simulink model "ACAC2024A"  (R2023b)
settings: Solver=ode23tb  StartTime=0.0  StopTime=0.3  FixedStep=1e-6  RelTol=1e-2
libraries: spsIGBTDiodeLib x8, spsSeriesRLCBranchLib x5, spsCurrentMeasurementLib x4, spsVoltageMeasurementLib x4, spsGroundLib x2, slpidlib x2, spsTriangleGeneratorLib x2, spsACVoltageSourceLib x1, sps_lib x1
settings Model: Creator=yaoya  LastModifiedBy=yaoya

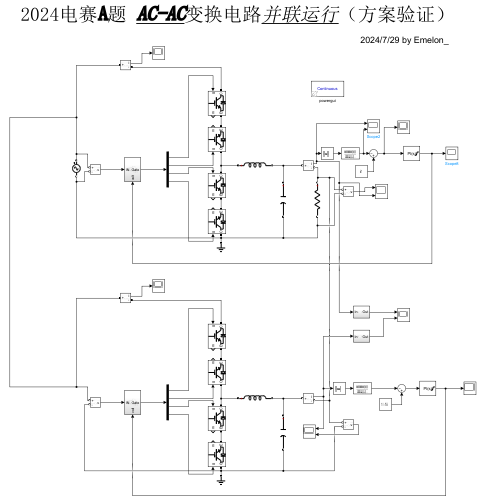
[thumbnail: Simulink's stored preview of the top-level diagram]
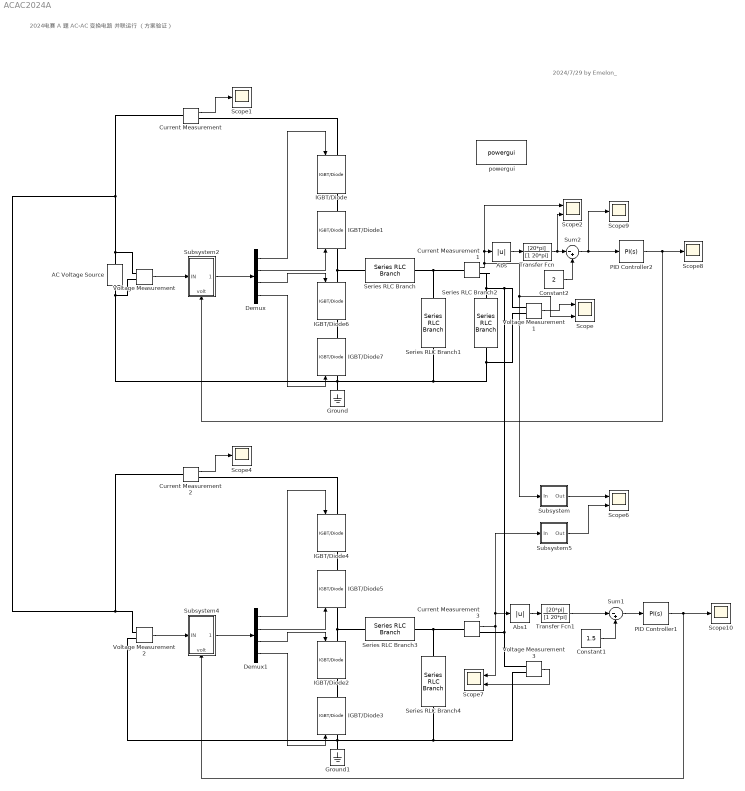
== system ACAC2024A ==
  note: 2024电赛 A 题 AC-AC 变换电路 并联运行 （方案验证）
  note: 2024/7/29 by Emelon_
  AC Voltage Source : spsACVoltageSourceLib/AC Voltage Source  Amplitude=100  Phase=0  Frequency=50  SampleTime=0  Measurements=None  BusType=swing  Pref=10e3  Qref=0  Qmin=-inf  Qmax=+inf
  Abs : Abs  SaturateOnIntegerOverflow=off
  Abs1 : Abs  SaturateOnIntegerOverflow=off
  Constant1 : Constant  Value=1.5
  Constant2 : Constant  Value=2
  Current Measurement{,1..3} (4 alike) : spsCurrentMeasurementLib/Current Measurement  PhasorSimulation=off  OutputType=Complex  PSBequivalent=0
  Demux : Demux
  Demux1 : Demux
  Ground : spsGroundLib/Ground  LConnTagsString=a
  Ground1 : spsGroundLib/Ground  LConnTagsString=a
  IGBT/Diode{,1..7} (8 alike) : spsIGBTDiodeLib/IGBT//Diode  Ron=1e-3  Rs=1e5  Cs=inf  Measurements=on
  PID Controller1 : slpidlib/PID Controller  Controller=PI  Form=Parallel  TimeDomain=Continuous-time  UseExternalTs=off  SampleTime=-1  IntegratorMethod=Forward Euler  FilterMethod=Forward Euler  ControllerParametersSource=internal  P=0.1  I=400  UseKiTs=off  D=10  N=100  UseFilter=on  TunerSelectOption=Transfer Function Based (PID Tuner App)  InitialConditionSource=internal  InitialConditionForIntegrator=0  InitialConditionForFilter=0  DifferentiatorICPrevScaledInput=0  ExternalReset=none  TrackingMode=off  Kt=1  LimitOutput=on  SatLimitsSource=internal  UpperSaturationLimit=30  LowerSaturationLimit=0  LinearizeAsGain=on  AntiWindupMode=none  Kb=1  LimitIntegrator=on  UpperIntegratorSaturationLimit=300  LowerIntegratorSaturationLimit=-300  POutMin=[]  POutMax=[]  IOutMin=[]  IOutMax=[]  DOutMin=[]  DOutMax=[]  NOutMin=[]  NOutMax=[]  SumOutMin=[]  SumOutMax=[]  SaturationOutMin=[]  SaturationOutMax=[]  PParamMin=[]  PParamMax=[]  IParamMin=[]  IParamMax=[]  DParamMin=[]  DParamMax=[]  NParamMin=[]  NParamMax=[]  KbParamMin=[]  KbParamMax=[]  KtParamMin=[]  KtParamMax=[]  KbOutMin=[]  KbOutMax=[]  KtOutMin=[]  KtOutMax=[]  IntegratorOutMin=[]  IntegratorOutMax=[]  FilterOutMin=[]  FilterOutMax=[]  SumI1OutMin=[]  SumI1OutMax=[]  SumI2OutMin=[]  SumI2OutMax=[]  SumI3OutMin=[]  SumI3OutMax=[]  SumI4OutMin=[]  SumI4OutMax=[]  SumDOutMin=[]  SumDOutMax=[]  DifferentiatorOutMin=[]  DifferentiatorOutMax=[]  FilterDiffOutCoefMin=[]  FilterDiffOutCoefMax=[]  ReciprocalOutMin=[]  ReciprocalOutMax=[]  SumDenOutMin=[]  SumDenOutMax=[]  SumNumOutMin=[]  SumNumOutMax=[]  DivideOutMin=[]  DivideOutMax=[]  UdiffTsProdOutMin=[]  UdiffTsProdOutMax=[]  NTsProdOutMin=[]  NTsProdOutMax=[]  UintegralTsProdOutMin=[]  UintegralTsProdOutMax=[]  UngainTsProdOutMin=[]  UngainTsProdOutMax=[]  ClampingZeroOutDataTypeStr=Inherit: Inherit via back propagation  ClampingZeroOutMin=[]  ClampingZeroOutMax=[]  FilterDenConstantOutDataTypeStr=Inherit: Inherit via back propagation  FilterDenConstantOutMin=[]  FilterDenConstantOutMax=[]  PCopyOutDataTypeStr=Inherit: Inherit via back propagation  PCopyOutMin=[]  PCopyOutMax=[]  NCopyOutDataTypeStr=Inherit: Inherit via back propagation  NCopyOutMin=[]  NCopyOutMax=[]  IntegratorContinuousStateAttributes=''  IntegratorStateMustResolveToSignalObject=off  IntegratorRTWStateStorageClass=Auto  FilterContinuousStateAttributes=''  FilterStateMustResolveToSignalObject=off  FilterRTWStateStorageClass=Auto  ParallelPVariant=InternalParameters  IdealPVariant=Disabled  IVariant=InternalParameters  DVariant=Disabled  IntegratorVariant=Continuous  SatVariant=Enabled  AWVariant=Passthrough  PCopyVariant=Disabled  TRVariant=Disabled  FdbkBlocksVariant=Forward  IdealPFdbkVariant=Disabled  SatFdbkVariant=Disabled  DerivativeFilterVariant=Disabled  NVariant=Disabled  NCopyVariant=Disabled_SignalSpec  FilterICVariant=Disabled  IntegratorICVariant=InternalICs  ExternalResetVariant=Disabled  TRSumVariant=Passthrough  SumFdbkVariant=Disabled  SumVariant=Sum_PI  TsampFilterVariant=InternalTs  TsampNgainVariant=Passthrough  TsampIntegralVariant=Disabled_SignalSpec  ExternalSaturationOutDataTypeStr=Inherit: Same as second input
  PID Controller2 : slpidlib/PID Controller  Controller=PI  Form=Parallel  TimeDomain=Continuous-time  UseExternalTs=off  SampleTime=-1  IntegratorMethod=Forward Euler  FilterMethod=Forward Euler  ControllerParametersSource=internal  P=0.1  I=400  UseKiTs=off  D=10  N=100  UseFilter=on  TunerSelectOption=Transfer Function Based (PID Tuner App)  InitialConditionSource=internal  InitialConditionForIntegrator=0  InitialConditionForFilter=0  DifferentiatorICPrevScaledInput=0  ExternalReset=none  TrackingMode=off  Kt=1  LimitOutput=on  SatLimitsSource=internal  UpperSaturationLimit=30  LowerSaturationLimit=0  LinearizeAsGain=on  AntiWindupMode=none  Kb=1  LimitIntegrator=on  UpperIntegratorSaturationLimit=300  LowerIntegratorSaturationLimit=-300  POutMin=[]  POutMax=[]  IOutMin=[]  IOutMax=[]  DOutMin=[]  DOutMax=[]  NOutMin=[]  NOutMax=[]  SumOutMin=[]  SumOutMax=[]  SaturationOutMin=[]  SaturationOutMax=[]  PParamMin=[]  PParamMax=[]  IParamMin=[]  IParamMax=[]  DParamMin=[]  DParamMax=[]  NParamMin=[]  NParamMax=[]  KbParamMin=[]  KbParamMax=[]  KtParamMin=[]  KtParamMax=[]  KbOutMin=[]  KbOutMax=[]  KtOutMin=[]  KtOutMax=[]  IntegratorOutMin=[]  IntegratorOutMax=[]  FilterOutMin=[]  FilterOutMax=[]  SumI1OutMin=[]  SumI1OutMax=[]  SumI2OutMin=[]  SumI2OutMax=[]  SumI3OutMin=[]  SumI3OutMax=[]  SumI4OutMin=[]  SumI4OutMax=[]  SumDOutMin=[]  SumDOutMax=[]  DifferentiatorOutMin=[]  DifferentiatorOutMax=[]  FilterDiffOutCoefMin=[]  FilterDiffOutCoefMax=[]  ReciprocalOutMin=[]  ReciprocalOutMax=[]  SumDenOutMin=[]  SumDenOutMax=[]  SumNumOutMin=[]  SumNumOutMax=[]  DivideOutMin=[]  DivideOutMax=[]  UdiffTsProdOutMin=[]  UdiffTsProdOutMax=[]  NTsProdOutMin=[]  NTsProdOutMax=[]  UintegralTsProdOutMin=[]  UintegralTsProdOutMax=[]  UngainTsProdOutMin=[]  UngainTsProdOutMax=[]  ClampingZeroOutDataTypeStr=Inherit: Inherit via back propagation  ClampingZeroOutMin=[]  ClampingZeroOutMax=[]  FilterDenConstantOutDataTypeStr=Inherit: Inherit via back propagation  FilterDenConstantOutMin=[]  FilterDenConstantOutMax=[]  PCopyOutDataTypeStr=Inherit: Inherit via back propagation  PCopyOutMin=[]  PCopyOutMax=[]  NCopyOutDataTypeStr=Inherit: Inherit via back propagation  NCopyOutMin=[]  NCopyOutMax=[]  IntegratorContinuousStateAttributes=''  IntegratorStateMustResolveToSignalObject=off  IntegratorRTWStateStorageClass=Auto  FilterContinuousStateAttributes=''  FilterStateMustResolveToSignalObject=off  FilterRTWStateStorageClass=Auto  ParallelPVariant=InternalParameters  IdealPVariant=Disabled  IVariant=InternalParameters  DVariant=Disabled  IntegratorVariant=Continuous  SatVariant=Enabled  AWVariant=Passthrough  PCopyVariant=Disabled  TRVariant=Disabled  FdbkBlocksVariant=Forward  IdealPFdbkVariant=Disabled  SatFdbkVariant=Disabled  DerivativeFilterVariant=Disabled  NVariant=Disabled  NCopyVariant=Disabled_SignalSpec  FilterICVariant=Disabled  IntegratorICVariant=InternalICs  ExternalResetVariant=Disabled  TRSumVariant=Passthrough  SumFdbkVariant=Disabled  SumVariant=Sum_PI  TsampFilterVariant=InternalTs  TsampNgainVariant=Passthrough  TsampIntegralVariant=Disabled_SignalSpec  ExternalSaturationOutDataTypeStr=Inherit: Same as second input
  Scope{,2,6..7} (4 alike) : Scope  NumInputPorts=2
  Scope{1,4,8..10} (5 alike) : Scope
  Series RLC Branch : spsSeriesRLCBranchLib/Series RLC Branch  LConnTagsString=__new0  RConnTagsString=__new0  BranchType=L  Resistance=1  Inductance=1e-3  SetiL0=off  InitialCurrent=0  Capacitance=1e-6  Setx0=off  InitialVoltage=0  Measurements=None
  Series RLC Branch1 : spsSeriesRLCBranchLib/Series RLC Branch  LConnTagsString=__new0  RConnTagsString=__new0  BranchType=C  Resistance=1  Inductance=1e-3  SetiL0=off  InitialCurrent=0  Capacitance=2e-5  Setx0=off  InitialVoltage=0  Measurements=None
  Series RLC Branch2 : spsSeriesRLCBranchLib/Series RLC Branch  LConnTagsString=__new0  RConnTagsString=__new0  BranchType=R  Resistance=2  Inductance=1e-3  SetiL0=off  InitialCurrent=0  Capacitance=1e-6  Setx0=off  InitialVoltage=0  Measurements=None
  Series RLC Branch3 : spsSeriesRLCBranchLib/Series RLC Branch  LConnTagsString=__new0  RConnTagsString=__new0  BranchType=L  Resistance=1  Inductance=1e-3  SetiL0=off  InitialCurrent=0  Capacitance=1e-6  Setx0=off  InitialVoltage=0  Measurements=None
  Series RLC Branch4 : spsSeriesRLCBranchLib/Series RLC Branch  LConnTagsString=__new0  RConnTagsString=__new0  BranchType=C  Resistance=1  Inductance=1e-3  SetiL0=off  InitialCurrent=0  Capacitance=2e-5  Setx0=off  InitialVoltage=0  Measurements=None
  Subsystem : Subsystem
  Subsystem2 : Subsystem
      settings: PortSchema="{\"entries\":[{\"content\":{\"sides\":[{\"content\":{\"connectorIds\":[\"In1\"]},\"type\":\"ConnectorPlacement.EquallySpacedRectSide\",\"uuid\":\"9bf67f15-6df5-49ec-9e97-b45d328a62b5\"},{\"content\":{\"connectorIds\":[\"Out1\"],\"side\":\"RIGHT\"},\"type\":\"ConnectorPlacement.EquallySpacedRectSide\",\"uuid\":\"3ba98dab-abca-4a9b-814d-0fc91b168aa2\"},{\"content\":{\"side\":\"TOP\"},\"type\":\"ConnectorPlacement.EquallySpacedRectSide\",\"uuid\":\"37cf702e-e048-48c7-bc32-8a6fb077cf42\"},{\"content\":{\"connectorIds\":[\"In2\"],\"side\":\"BOTTOM\"},\"type\":\"ConnectorPlacement.EquallySpacedRectSide\",\"uuid\":\"a7b4d778-482e-4954-b60e-282dd71c48e8\"}]},\"type\":\"ConnectorPlacement.EquallySpacedConnector\",\"uuid\":\"958a7cd0-394f-4262-9a45-8e78109bd1aa\"}],\"packageUris\":[\"http://schema.mathworks.com/mf0/Connector/R2020b\"],\"version\":\"1.0\"}"
  Subsystem4 : Subsystem
      settings: PortSchema="{\"entries\":[{\"content\":{\"sides\":[{\"content\":{\"connectorIds\":[\"In1\"]},\"type\":\"ConnectorPlacement.EquallySpacedRectSide\",\"uuid\":\"9bf67f15-6df5-49ec-9e97-b45d328a62b5\"},{\"content\":{\"connectorIds\":[\"Out1\"],\"side\":\"RIGHT\"},\"type\":\"ConnectorPlacement.EquallySpacedRectSide\",\"uuid\":\"3ba98dab-abca-4a9b-814d-0fc91b168aa2\"},{\"content\":{\"side\":\"TOP\"},\"type\":\"ConnectorPlacement.EquallySpacedRectSide\",\"uuid\":\"37cf702e-e048-48c7-bc32-8a6fb077cf42\"},{\"content\":{\"connectorIds\":[\"In2\"],\"side\":\"BOTTOM\"},\"type\":\"ConnectorPlacement.EquallySpacedRectSide\",\"uuid\":\"a7b4d778-482e-4954-b60e-282dd71c48e8\"}]},\"type\":\"ConnectorPlacement.EquallySpacedConnector\",\"uuid\":\"958a7cd0-394f-4262-9a45-8e78109bd1aa\"}],\"packageUris\":[\"http://schema.mathworks.com/mf0/Connector/R2020b\"],\"version\":\"1.0\"}"
  Subsystem5 : Subsystem
  Sum1 : Sum  Inputs=|-+
  Sum2 : Sum  Inputs=|-+
  Transfer Fcn : TransferFcn  Numerator=[20*pi]  Denominator=[1 20*pi]
  Transfer Fcn1 : TransferFcn  Numerator=[20*pi]  Denominator=[1 20*pi]
  Voltage Measurement{,1..3} (4 alike) : spsVoltageMeasurementLib/Voltage Measurement  PhasorSimulation=off  OutputType=Complex  PSBequivalent=0
  powergui : sps_lib/powergui  Priority=1  SimulationMode=Continuous  SampleTime=50e-6  frequency=60  Iterations=50  frequencyindice=50  Pbase=100e6  ErrMax=1e-4  UnitsV=kV  UnitsW=MW  buscounter=0  FunctionMessages=off  echomessages=off  EnableUseOfTLC=off  CurrentSourceSwitches=off  DisableSnubberDevices=off  DisableRonSwitches=off  DisableVfSwitches=off  DisplayEquations=off  AutomaticDiscreteSolvers=off  SolverType=Tustin/Backward Euler (TBE)  Interpol=off  ExternalGateDelay=off  methode=off  Ts=100  x0status=blocks  SPID=on  SwTol=0  HookPort=off  NonlinearTolerance=1e-4  nMaxIteration=100  ContinueOnMaxIteration=off  RestoreLinks=warning  ResistiveCurrentMeasurement=off  Frange=[0:2:500]  Ylog=off  Xlog=on  ShowGrid=off  save=off  variable=ZData  structure=0  ZoomFFT=off  StartTime=0.0  cycles=1  DisplayStyle=1  fundamental=60  FreqAxis=off  MaxFrequency=1000  frequencyindicesteady=1  RmsSteady=1  display=off
  wires:
  Demux/1 -> IGBT/Diode/1
  Demux/2 -> IGBT/Diode1/1
  Current Measurement/1 -> Scope1/1
  Voltage Measurement/1 -> Subsystem2/1(IN)
  Subsystem2/1(Gate) -> Demux/1
  Current Measurement1/1 -> Scope/2, Subsystem/1(In), Abs/1, Scope2/1
  PID Controller1/1 -> Scope10/1, Subsystem4/2(volt)
  Constant1/1 -> Sum1/2
  Sum1/1 -> PID Controller1/1
  Current Measurement3/1 -> Subsystem5/1(In), Abs1/1, Scope7/1
  Subsystem4/1(Gate) -> Demux1/1
  Voltage Measurement2/1 -> Subsystem4/1(IN)
  Current Measurement2/1 -> Scope4/1
  Voltage Measurement3/1 -> Scope7/2
  Demux1/2 -> IGBT/Diode5/1
  Demux1/1 -> IGBT/Diode4/1
  Demux1/3 -> IGBT/Diode2/1
  Demux1/4 -> IGBT/Diode3/1
  Demux/3 -> IGBT/Diode6/1
  Demux/4 -> IGBT/Diode7/1
  PID Controller2/1 -> Scope8/1, Subsystem2/2(volt)
  Sum2/1 -> Scope9/1, PID Controller2/1
  Constant2/1 -> Sum2/2
  Abs/1 -> Transfer Fcn/1
  Transfer Fcn/1 -> Scope2/2, Sum2/1
  Voltage Measurement1/1 -> Scope/1
  Abs1/1 -> Transfer Fcn1/1
  Transfer Fcn1/1 -> Sum1/1
  Subsystem/1(Out) -> Scope6/1
  Subsystem5/1(Out) -> Scope6/2
  connections:
  IGBT/Diode1/RConn1 -- IGBT/Diode/RConn1
  Ground/LConn1 -- Voltage Measurement/LConn2 -- AC Voltage Source/LConn1 -- Voltage Measurement1/LConn2 -- Series RLC Branch2/RConn1 -- Series RLC Branch1/RConn1 -- IGBT/Diode7/LConn1
  Series RLC Branch1/LConn1 -- Current Measurement1/LConn1 -- Series RLC Branch/RConn1
  Current Measurement2/LConn1 -- Voltage Measurement2/LConn1 -- AC Voltage Source/RConn1 -- Voltage Measurement/LConn1 -- Current Measurement/LConn1
  Current Measurement/RConn1 -- IGBT/Diode/LConn1
  Series RLC Branch2/LConn1 -- Current Measurement3/RConn1 -- Voltage Measurement3/LConn1 -- Voltage Measurement1/LConn1 -- Current Measurement1/RConn1
  IGBT/Diode5/LConn1 -- IGBT/Diode2/LConn1 -- Series RLC Branch3/LConn1
  Voltage Measurement2/LConn2 -- IGBT/Diode3/LConn1 -- Ground1/LConn1 -- Voltage Measurement3/LConn2 -- Series RLC Branch4/RConn1
  Current Measurement3/LConn1 -- Series RLC Branch4/LConn1 -- Series RLC Branch3/RConn1
  Current Measurement2/RConn1 -- IGBT/Diode4/LConn1
  IGBT/Diode5/RConn1 -- IGBT/Diode4/RConn1
  Series RLC Branch/LConn1 -- IGBT/Diode6/LConn1 -- IGBT/Diode1/LConn1
  IGBT/Diode3/RConn1 -- IGBT/Diode2/RConn1
  IGBT/Diode7/RConn1 -- IGBT/Diode6/RConn1

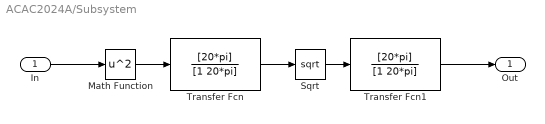
== system ACAC2024A/Subsystem ==
  In : Inport
  Math Function : Math  Operator=square
  Sqrt : Sqrt
  Transfer Fcn : TransferFcn  Numerator=[20*pi]  Denominator=[1 20*pi]
  Transfer Fcn1 : TransferFcn  Numerator=[20*pi]  Denominator=[1 20*pi]
  Out : Outport
  wires:
  In/1 -> Math Function/1
  Transfer Fcn/1 -> Sqrt/1
  Math Function/1 -> Transfer Fcn/1
  Sqrt/1 -> Transfer Fcn1/1
  Transfer Fcn1/1 -> Out/1

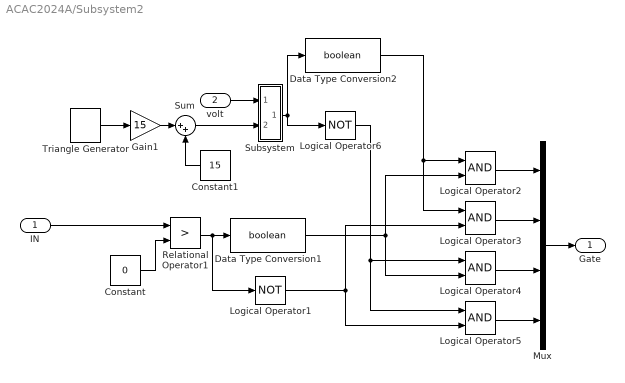
== system ACAC2024A/Subsystem2 ==
  IN : Inport
  volt : Inport  Port=2
  Constant : Constant  Value=0
  Constant1 : Constant  Value=15
  Data Type Conversion1 : DataTypeConversion  OutDataTypeStr=boolean  SaturateOnIntegerOverflow=off  RndMeth=Floor
  Data Type Conversion2 : DataTypeConversion  OutDataTypeStr=boolean  SaturateOnIntegerOverflow=off  RndMeth=Floor
  Gain1 : Gain  Gain=15
  Logical Operator1 : Logic  Operator=NOT  AllPortsSameDT=off  OutDataTypeStr=boolean
  Logical Operator{2..5} (4 alike) : Logic  AllPortsSameDT=off  OutDataTypeStr=boolean
  Logical Operator6 : Logic  Operator=NOT  AllPortsSameDT=off  OutDataTypeStr=boolean
  Mux : Mux
  Relational Operator1 : RelationalOperator  Operator=>  OutDataTypeStr=boolean  RndMeth=Simplest  InputSameDT=off
  Subsystem : Subsystem
  Sum : Sum  Inputs=|++
  Triangle Generator : spsTriangleGeneratorLib/Triangle Generator  Freq=1e4  Phase=90  Ts=0
  Gate : Outport
  wires:
  Subsystem/1(out) -> Data Type Conversion2/1, Logical Operator6/1
  Logical Operator6/1 -> Logical Operator5/1, Logical Operator4/1
  Logical Operator2/1 -> Mux/1
  Data Type Conversion1/1 -> Logical Operator4/2, Logical Operator2/2
  IN/1 -> Relational Operator1/1
  Triangle Generator/1 -> Gain1/1
  Mux/1 -> Gate/1
  Logical Operator1/1 -> Logical Operator3/2, Logical Operator5/2
  Gain1/1 -> Sum/1
  Relational Operator1/1 -> Logical Operator1/1, Data Type Conversion1/1
  Data Type Conversion2/1 -> Logical Operator3/1, Logical Operator2/1
  Sum/1 -> Subsystem/2(-)
  Logical Operator5/1 -> Mux/4
  Logical Operator4/1 -> Mux/3
  Logical Operator3/1 -> Mux/2
  Constant/1 -> Relational Operator1/2
  Constant1/1 -> Sum/2
  volt/1 -> Subsystem/1(+)

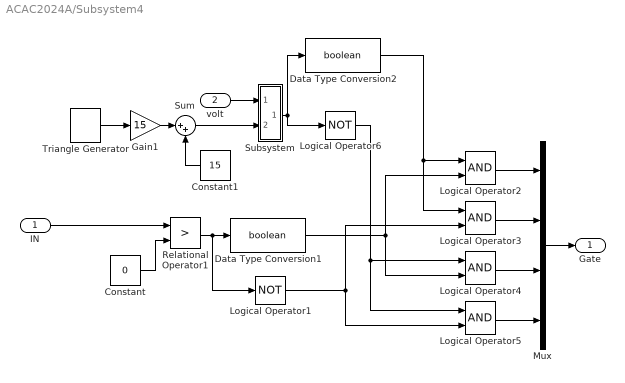
== system ACAC2024A/Subsystem4 ==
  IN : Inport
  volt : Inport  Port=2
  Constant : Constant  Value=0
  Constant1 : Constant  Value=15
  Data Type Conversion1 : DataTypeConversion  OutDataTypeStr=boolean  SaturateOnIntegerOverflow=off  RndMeth=Floor
  Data Type Conversion2 : DataTypeConversion  OutDataTypeStr=boolean  SaturateOnIntegerOverflow=off  RndMeth=Floor
  Gain1 : Gain  Gain=15
  Logical Operator1 : Logic  Operator=NOT  AllPortsSameDT=off  OutDataTypeStr=boolean
  Logical Operator{2..5} (4 alike) : Logic  AllPortsSameDT=off  OutDataTypeStr=boolean
  Logical Operator6 : Logic  Operator=NOT  AllPortsSameDT=off  OutDataTypeStr=boolean
  Mux : Mux
  Relational Operator1 : RelationalOperator  Operator=>  OutDataTypeStr=boolean  RndMeth=Simplest  InputSameDT=off
  Subsystem : Subsystem
  Sum : Sum  Inputs=|++
  Triangle Generator : spsTriangleGeneratorLib/Triangle Generator  Freq=1e4  Phase=90  Ts=0
  Gate : Outport
  wires:
  volt/1 -> Subsystem/1(+)
  Constant1/1 -> Sum/2
  Constant/1 -> Relational Operator1/2
  Logical Operator3/1 -> Mux/2
  Logical Operator4/1 -> Mux/3
  Logical Operator5/1 -> Mux/4
  Sum/1 -> Subsystem/2(-)
  Data Type Conversion2/1 -> Logical Operator2/1, Logical Operator3/1
  Relational Operator1/1 -> Data Type Conversion1/1, Logical Operator1/1
  Gain1/1 -> Sum/1
  Logical Operator1/1 -> Logical Operator5/2, Logical Operator3/2
  Mux/1 -> Gate/1
  Triangle Generator/1 -> Gain1/1
  IN/1 -> Relational Operator1/1
  Data Type Conversion1/1 -> Logical Operator2/2, Logical Operator4/2
  Logical Operator2/1 -> Mux/1
  Logical Operator6/1 -> Logical Operator4/1, Logical Operator5/1
  Subsystem/1(out) -> Logical Operator6/1, Data Type Conversion2/1

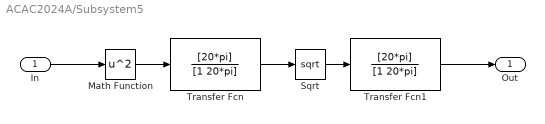
== system ACAC2024A/Subsystem5 ==
  In : Inport
  Math Function : Math  Operator=square
  Sqrt : Sqrt
  Transfer Fcn : TransferFcn  Numerator=[20*pi]  Denominator=[1 20*pi]
  Transfer Fcn1 : TransferFcn  Numerator=[20*pi]  Denominator=[1 20*pi]
  Out : Outport
  wires:
  Transfer Fcn1/1 -> Out/1
  Sqrt/1 -> Transfer Fcn1/1
  Math Function/1 -> Transfer Fcn/1
  Transfer Fcn/1 -> Sqrt/1
  In/1 -> Math Function/1

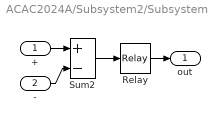
== system ACAC2024A/Subsystem2/Subsystem ==
  + : Inport
  - : Inport  Port=2
  Relay : Relay  OnSwitchValue=0.05  OffSwitchValue=-0.05
  Sum2 : Sum  Inputs=|+-
  out : Outport
  wires:
  Sum2/1 -> Relay/1
  Relay/1 -> out/1
  +/1 -> Sum2/1
  -/1 -> Sum2/2

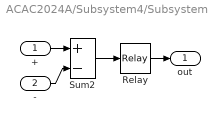
== system ACAC2024A/Subsystem4/Subsystem ==
  + : Inport
  - : Inport  Port=2
  Relay : Relay  OnSwitchValue=0.05  OffSwitchValue=-0.05
  Sum2 : Sum  Inputs=|+-
  out : Outport
  wires:
  -/1 -> Sum2/2
  +/1 -> Sum2/1
  Relay/1 -> out/1
  Sum2/1 -> Relay/1
